simulink model "cob4_5"  (R2016a)
settings: Solver=FixedStepAuto  StartTime=0.0  StopTime=100  FixedStep=0.01  RelTol=1e-3
undefined symbols (not defined in the file): a, a2, arm_config, arm_link1, DiscIntNeverNeededParam, gripper_link, j, n, shoulder1_link, shoulder2_link, torso_link, X, Y, Z
libraries: sm_lib x81, nesl_utility x42, roblocks x3
(part 1 of 2)
settings Model: Creator=bbrito  LastModifiedBy=root

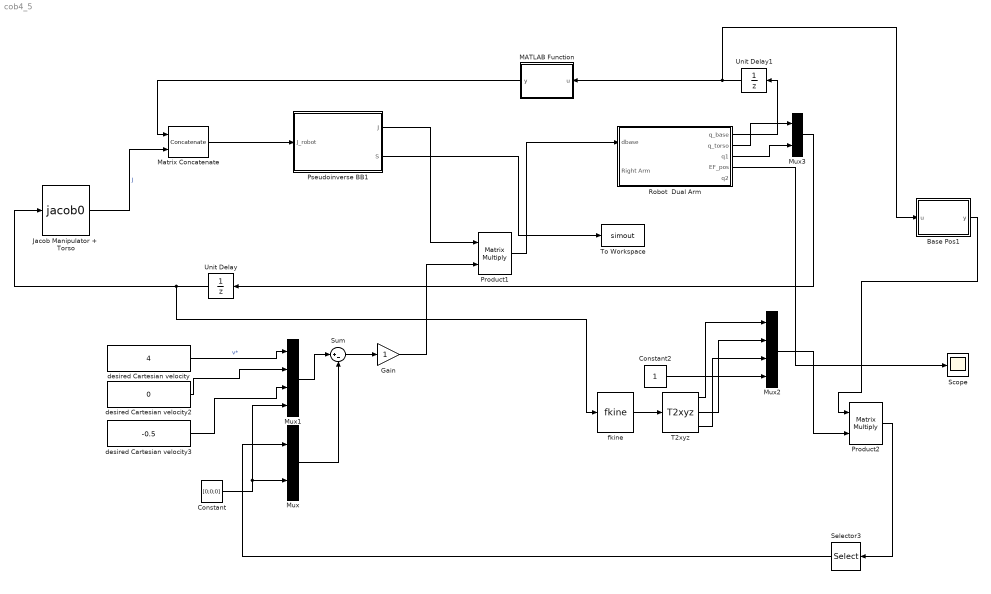
== system cob4_5 ==
  Base Pos1 : MATLAB Function  TreatAsAtomicUnit=on  mask{torso_link=torso_link}
      mask prompts: torso_link "Torso LInk"
  Constant : Constant  Value=[0;0;0]  SampleTime=-1
  Constant2 : Constant  SampleTime=-1
  Gain : Gain
  "Jacob Manipulator +  Torso " : roblocks/Kinematics/jacob0   robot=robot
  MATLAB Function : MATLAB Function  TreatAsAtomicUnit=on
  Matrix Concatenate : Concatenate  Mode=Multidimensional array  ConcatenateDimension=2
  Mux : Mux  Inputs=2
  Mux1 : Mux
  Mux2 : Mux
  Mux3 : Mux  Inputs=2
  Product1 : Product  Multiplication=Matrix(*)  SaturateOnIntegerOverflow=on  OutDataTypeStr=Inherit: Same as first input
  Product2 : Product  Multiplication=Matrix(*)  SaturateOnIntegerOverflow=on  OutDataTypeStr=Inherit: Same as first input
  Pseudoinverse BB1 : MATLAB Function  TreatAsAtomicUnit=on  mask{dim=[n(1)+4 6]}
      mask prompts: dim "Jacobian Dimensions"
  Robot  Dual Arm : Subsystem  TreatAsAtomicUnit=on
  Scope : Scope
  Selector3 : Selector  InputPortWidth=4  IndexOptions=Index vector (dialog)  Indices=[1:3]  OutputSizes=1
  Sum : Sum  Inputs=|+-
  T2xyz : roblocks/Transform Conversion/T2xyz
  To Workspace : ToWorkspace  VariableName=simout  SaveFormat=Structure  SampleTime=-1
  Unit Delay : UnitDelay  InitialCondition=zeros(n(1)+2,1)  SampleTime=-1
  Unit Delay1 : UnitDelay  InitialCondition=zeros(2,1)  SampleTime=-1
  desired Cartesian velocity : Constant  Value=4  VectorParams1D=off  SampleTime=-1
  desired Cartesian velocity2 : Constant  Value=0  VectorParams1D=off  SampleTime=-1
  desired Cartesian velocity3 : Constant  Value=-0.5  VectorParams1D=off  SampleTime=-1
  fkine : roblocks/Kinematics/fkine  robot=robot
  wires:
  fkine/1 -> T2xyz/1
  Sum/1 -> Gain/1
  Mux/1 -> Sum/2
  T2xyz/1 -> Mux2/1
  Robot  Dual Arm/3(q1) -> Mux3/2
  Constant/1 -> Mux/2, Mux1/4
  T2xyz/3 -> Mux2/3
  T2xyz/2 -> Mux2/2
  desired Cartesian velocity/1 -> Mux1/1  "v*"
  Mux1/1 -> Sum/1
  Constant2/1 -> Mux2/4
  desired Cartesian velocity2/1 -> Mux1/2
  desired Cartesian velocity3/1 -> Mux1/3
  Mux2/1 -> Product2/2
  "Jacob Manipulator +  Torso "/1 -> Matrix Concatenate/2  "J"
  Matrix Concatenate/1 -> Pseudoinverse BB1/1(J_robot)
  MATLAB Function/1(y) -> Matrix Concatenate/1
  Base Pos1/1(y) -> Product2/1
  Product2/1 -> Selector3/1
  Selector3/1 -> Mux/1
  Pseudoinverse BB1/1(J) -> Product1/1
  Gain/1 -> Product1/2
  Robot  Dual Arm/2(q_torso) -> Mux3/1
  Unit Delay/1 -> fkine/1, "Jacob Manipulator +  Torso "/1
  Mux3/1 -> Unit Delay/1
  Robot  Dual Arm/1(q_base) -> Unit Delay1/1
  Unit Delay1/1 -> Base Pos1/1(u), MATLAB Function/1(u)
  Product1/1 -> Robot  Dual Arm/1(dbase)
  Robot  Dual Arm/4(EF_pos) -> Scope/1
  Pseudoinverse BB1/2(S) -> To Workspace/1

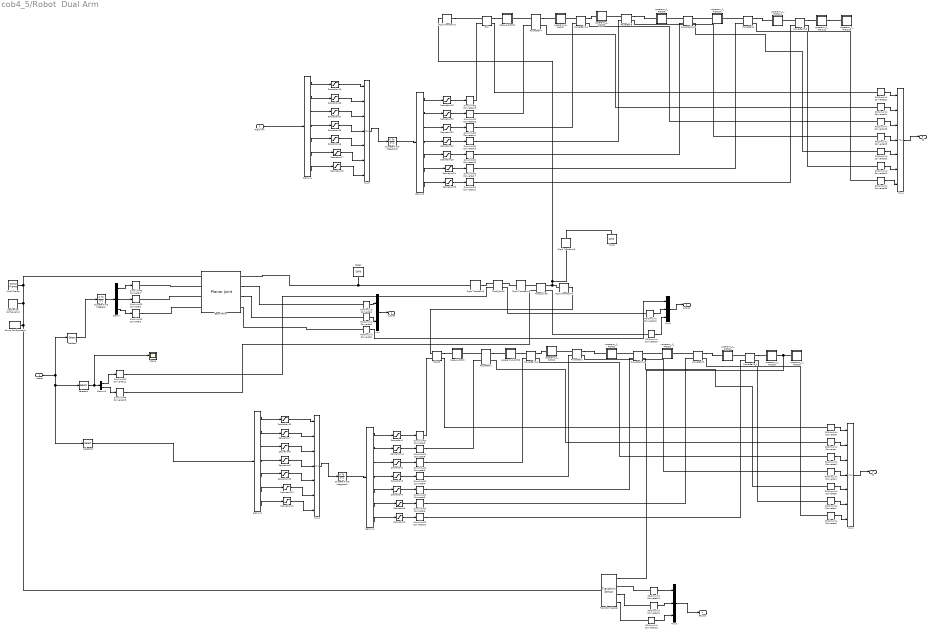
== system cob4_5/Robot  Dual Arm ==
  dbase : Inport
  Right Arm : Inport  Port=2
  Base Motion : sm_lib/Joints/Planar Joint  SenseConstraintForce=off  SenseConstraintForceX=off  SenseConstraintForceY=off  SenseConstraintForceZ=off  SenseConstraintTorque=off  SenseConstraintTorqueX=off  SenseConstraintTorqueY=off  SenseConstraintTorqueZ=off  SenseTotalForce=off  SenseTotalForceX=off  SenseTotalForceY=off  SenseTotalForceZ=off  SenseTotalTorque=off  SenseTotalTorqueX=off  SenseTotalTorqueY=off  SenseTotalTorqueZ=off  CompositeWrenchDir=FollowerOnBase  CompositeWrenchFrame=BaseFrame  PxEquilibriumPosition=0  PxEquilibriumPositionUnits=m  PxSpringStiffness=0  PxSpringStiffnessUnits=N/m  PxDampingCoefficient=0  PxDampingCoefficientUnits=N/(m/s)  PxTorqueActuationMode=ComputedTorque  PxMotionActuationMode=InputMotion  PxSensePosition=on  PxSenseVelocity=off  PxSenseAcceleration=off  PxSenseTorqueForce=off  PxPositionTargetSpecify=off  PxPositionTargetPriority=High  PxPositionTargetValue=0  PxPositionTargetValueUnits=m  PxVelocityTargetSpecify=off  PxVelocityTargetPriority=High  PxVelocityTargetValue=0  PxVelocityTargetValueUnits=m/s  PyEquilibriumPosition=0  PyEquilibriumPositionUnits=m  PySpringStiffness=0  PySpringStiffnessUnits=N/m  PyDampingCoefficient=0  PyDampingCoefficientUnits=N/(m/s)  PyTorqueActuationMode=ComputedTorque  PyMotionActuationMode=InputMotion  PySensePosition=on  PySenseVelocity=off  PySenseAcceleration=off  PySenseTorqueForce=off  PyPositionTargetSpecify=off  PyPositionTargetPriority=High  PyPositionTargetValue=0  PyPositionTargetValueUnits=m  PyVelocityTargetSpecify=off  PyVelocityTargetPriority=High  PyVelocityTargetValue=0  PyVelocityTargetValueUnits=m/s  RzEquilibriumPosition=0  RzEquilibriumPositionUnits=deg  RzSpringStiffness=0  RzSpringStiffnessUnits=N*m/deg  RzDampingCoefficient=0  RzDampingCoefficientUnits=N*m/(deg/s)  RzTorqueActuationMode=ComputedTorque  RzMotionActuationMode=InputMotion  RzSensePosition=on  RzSenseVelocity=off  RzSenseAcceleration=off  RzSenseTorqueForce=off  RzPositionTargetSpecify=off  RzPositionTargetPriority=High  RzPositionTargetValue=0  RzPositionTargetValueUnits=deg  RzVelocityTargetSpecify=off  RzVelocityTargetPriority=High  RzVelocityTargetValue=0  RzVelocityTargetValueUnits=deg/s
  Base1 : sm_lib/Body Elements/Solid  InertiaType=Custom  Mass=50  MassUnits=kg  CenterOfMass=[0 0 0]  CenterOfMassUnits=m  MomentsOfInertia=[5.652232699207 5.669473158652 3.683196351726]  MomentsOfInertiaUnits=kg*m^2  ProductsOfInertia=[-0.009719934438 1.293988226423 -0.007379583694]  ProductsOfInertiaUnits=kg*m^2  DensityBased=on  Density=1000  DensityUnits=kg/(m^3)  DoExposeReferenceFrame=on  SerializedFrames=<Frames/>  GraphicType=FromGeometry  MarkerShape=Sphere  MarkerSize=10  GraphicVisPropType=SimpleVisualProperties  GraphicDiffuseColor=[0.5 0.5 0.5]  GraphicSpecularColor=[0.5 0.5 0.5 1.0]  GraphicAmbientColor=[0.15 0.15 0.15 1.0]  GraphicEmissiveColor=[0.0 0.0 0.0 1.0]  GraphicShininess=75  GraphicOpacity=1.0  GeometryShape=FromFile  RectangleSize=[1 1]  RectangleSizeUnits=m  BrickDimensions=[1 1 1]  BrickDimensionUnits=m  CylinderRadius=1  CylinderRadiusUnits=m  CylinderLength=1  CylinderLengthUnits=m  SphereRadius=1  SphereRadiusUnits=m  EllipsoidRadii=[1 1 1]  EllipsoidRadiiUnits=m  ExtrusionCrossSection=[1 1; -1 1; -1 -1; 1 -1]  ExtrusionCrossSectionUnits=m  ExtrusionLength=1  ExtrusionLengthUnits=m  PolygonNumSides=3  PolygonOuterRadius=1  PolygonOuterRadiusUnits=m  ExtGeomFileType=STL  ExtGeomFileName=/home/bbrito/schunk_sim/base.stl  ExtGeomFileUnits=m  RevolutionCrossSection=[1 1; 1 -1; 2 -1; 2 1]  RevolutionCrossSectionUnits=m  RevolutionExtent=Full  RevolutionAngle=180  RevolutionAngleUnits=deg
  DL1 : sm_lib/Joints/Revolute Joint  SenseConstraintForce=off  SenseConstraintForceX=off  SenseConstraintForceY=off  SenseConstraintForceZ=off  SenseConstraintTorque=off  SenseConstraintTorqueX=off  SenseConstraintTorqueY=off  SenseConstraintTorqueZ=off  SenseTotalForce=off  SenseTotalForceX=off  SenseTotalForceY=off  SenseTotalForceZ=off  SenseTotalTorque=off  SenseTotalTorqueX=off  SenseTotalTorqueY=off  SenseTotalTorqueZ=off  CompositeWrenchDir=FollowerOnBase  CompositeWrenchFrame=BaseFrame  EquilibriumPosition=0  EquilibriumPositionUnits=deg  SpringStiffness=0  SpringStiffnessUnits=N*m/deg  DampingCoefficient=0  DampingCoefficientUnits=N*m/(deg/s)  TorqueActuationMode=ComputedTorque  MotionActuationMode=InputMotion  SensePosition=on  SenseVelocity=off  SenseAcceleration=off  SenseTorqueForce=off  PositionTargetSpecify=on  PositionTargetPriority=High  PositionTargetValue=0  PositionTargetValueUnits=deg  VelocityTargetSpecify=on  VelocityTargetPriority=High  VelocityTargetValue=0  VelocityTargetValueUnits=deg/s
  DL100 : sm_lib/Joints/Revolute Joint  SenseConstraintForce=off  SenseConstraintForceX=off  SenseConstraintForceY=off  SenseConstraintForceZ=off  SenseConstraintTorque=off  SenseConstraintTorqueX=off  SenseConstraintTorqueY=off  SenseConstraintTorqueZ=off  SenseTotalForce=off  SenseTotalForceX=off  SenseTotalForceY=off  SenseTotalForceZ=off  SenseTotalTorque=off  SenseTotalTorqueX=off  SenseTotalTorqueY=off  SenseTotalTorqueZ=off  CompositeWrenchDir=FollowerOnBase  CompositeWrenchFrame=BaseFrame  EquilibriumPosition=0  EquilibriumPositionUnits=deg  SpringStiffness=0  SpringStiffnessUnits=N*m/deg  DampingCoefficient=0  DampingCoefficientUnits=N*m/(deg/s)  TorqueActuationMode=ComputedTorque  MotionActuationMode=InputMotion  SensePosition=on  SenseVelocity=off  SenseAcceleration=off  SenseTorqueForce=off  PositionTargetSpecify=on  PositionTargetPriority=High  PositionTargetValue=0  PositionTargetValueUnits=deg  VelocityTargetSpecify=on  VelocityTargetPriority=High  VelocityTargetValue=0  VelocityTargetValueUnits=deg/s
  Demux : Demux  Outputs=3
  Demux{1..4} (4 alike) : Demux  Outputs=n(1)-1
  Demux5 : Demux  Outputs=2
  Discrete-Time Integrator : DiscreteIntegrator  InitialCondition=[0;0;0]  InitialConditionSetting=State (most efficient)  SampleTime=-1  ICPrevOutput=DiscIntNeverNeededParam  ICPrevScaledInput=DiscIntNeverNeededParam
  Discrete-Time Integrator1 : DiscreteIntegrator  InitialCondition=zeros(n(1)-1,1)  InitialConditionSetting=State (most efficient)  SampleTime=-1  ICPrevOutput=DiscIntNeverNeededParam  ICPrevScaledInput=DiscIntNeverNeededParam
  Discrete-Time Integrator3 : DiscreteIntegrator  InitialCondition=zeros(n(1)-1,1)  InitialConditionSetting=State (most efficient)  SampleTime=-1  ICPrevOutput=DiscIntNeverNeededParam  ICPrevScaledInput=DiscIntNeverNeededParam
  Mechanism Configuration : sm_lib/Utilities/Mechanism Configuration  UniformGravity=Constant  GravityVector=[0 0 -9.81]  GravityUnits=m/s^2  LinearizationDelta=0.01
  Mux : Mux  Inputs=2
  Mux{1..2,4..5} (4 alike) : Mux  Inputs=n(1)-1
  Mux3 : Mux  Inputs=3
  Mux6 : Mux  Inputs=3
  PS-Simulink Converter{,1..15,18..23} (22 alike) : nesl_utility/PS-Simulink Converter  PhysicalDomain=network_engine_domain  SubClassName=ps_output  LeftPortType=input  RightPortType=output  PseudoPeriodic=off  Frequencies=[]  Unit=1  AffineConversion=off
  PowerBall{1..6} (6 alike) : sm_lib/Joints/Revolute Joint  SenseConstraintForce=off  SenseConstraintForceX=off  SenseConstraintForceY=off  SenseConstraintForceZ=off  SenseConstraintTorque=off  SenseConstraintTorqueX=off  SenseConstraintTorqueY=off  SenseConstraintTorqueZ=off  SenseTotalForce=off  SenseTotalForceX=off  SenseTotalForceY=off  SenseTotalForceZ=off  SenseTotalTorque=off  SenseTotalTorqueX=off  SenseTotalTorqueY=off  SenseTotalTorqueZ=off  CompositeWrenchDir=FollowerOnBase  CompositeWrenchFrame=BaseFrame  EquilibriumPosition=0  EquilibriumPositionUnits=deg  SpringStiffness=0  SpringStiffnessUnits=N*m/deg  DampingCoefficient=0  DampingCoefficientUnits=N*m/(deg/s)  TorqueActuationMode=ComputedTorque  MotionActuationMode=InputMotion  SensePosition=on  SenseVelocity=off  SenseAcceleration=off  SenseTorqueForce=off  PositionTargetSpecify=on  PositionTargetPriority=High  PositionTargetValue=0  PositionTargetValueUnits=deg  VelocityTargetSpecify=on  VelocityTargetPriority=High  VelocityTargetValue=0  VelocityTargetValueUnits=deg/s
  PowerBall1_1 : sm_lib/Joints/Revolute Joint  SenseConstraintForce=off  SenseConstraintForceX=off  SenseConstraintForceY=off  SenseConstraintForceZ=off  SenseConstraintTorque=off  SenseConstraintTorqueX=off  SenseConstraintTorqueY=off  SenseConstraintTorqueZ=off  SenseTotalForce=off  SenseTotalForceX=off  SenseTotalForceY=off  SenseTotalForceZ=off  SenseTotalTorque=off  SenseTotalTorqueX=off  SenseTotalTorqueY=off  SenseTotalTorqueZ=off  CompositeWrenchDir=FollowerOnBase  CompositeWrenchFrame=BaseFrame  EquilibriumPosition=0  EquilibriumPositionUnits=deg  SpringStiffness=0  SpringStiffnessUnits=N*m/deg  DampingCoefficient=0  DampingCoefficientUnits=N*m/(deg/s)  TorqueActuationMode=ComputedTorque  MotionActuationMode=InputMotion  SensePosition=on  SenseVelocity=off  SenseAcceleration=off  SenseTorqueForce=off  PositionTargetSpecify=on  PositionTargetPriority=High  PositionTargetValue=0  PositionTargetValueUnits=deg  VelocityTargetSpecify=on  VelocityTargetPriority=High  VelocityTargetValue=0  VelocityTargetValueUnits=deg/s
  PowerBall1_2 : sm_lib/Joints/Revolute Joint  SenseConstraintForce=off  SenseConstraintForceX=off  SenseConstraintForceY=off  SenseConstraintForceZ=off  SenseConstraintTorque=off  SenseConstraintTorqueX=off  SenseConstraintTorqueY=off  SenseConstraintTorqueZ=off  SenseTotalForce=off  SenseTotalForceX=off  SenseTotalForceY=off  SenseTotalForceZ=off  SenseTotalTorque=off  SenseTotalTorqueX=off  SenseTotalTorqueY=off  SenseTotalTorqueZ=off  CompositeWrenchDir=FollowerOnBase  CompositeWrenchFrame=BaseFrame  EquilibriumPosition=0  EquilibriumPositionUnits=deg  SpringStiffness=0  SpringStiffnessUnits=N*m/deg  DampingCoefficient=0  DampingCoefficientUnits=N*m/(deg/s)  TorqueActuationMode=ComputedTorque  MotionActuationMode=InputMotion  SensePosition=on  SenseVelocity=off  SenseAcceleration=off  SenseTorqueForce=off  PositionTargetSpecify=on  PositionTargetPriority=High  PositionTargetValue=0  PositionTargetValueUnits=deg  VelocityTargetSpecify=on  VelocityTargetPriority=High  VelocityTargetValue=0  VelocityTargetValueUnits=deg/s
  PowerBall2_1 : sm_lib/Joints/Revolute Joint  SenseConstraintForce=off  SenseConstraintForceX=off  SenseConstraintForceY=off  SenseConstraintForceZ=off  SenseConstraintTorque=off  SenseConstraintTorqueX=off  SenseConstraintTorqueY=off  SenseConstraintTorqueZ=off  SenseTotalForce=off  SenseTotalForceX=off  SenseTotalForceY=off  SenseTotalForceZ=off  SenseTotalTorque=off  SenseTotalTorqueX=off  SenseTotalTorqueY=off  SenseTotalTorqueZ=off  CompositeWrenchDir=FollowerOnBase  CompositeWrenchFrame=BaseFrame  EquilibriumPosition=0  EquilibriumPositionUnits=deg  SpringStiffness=0  SpringStiffnessUnits=N*m/deg  DampingCoefficient=0  DampingCoefficientUnits=N*m/(deg/s)  TorqueActuationMode=ComputedTorque  MotionActuationMode=InputMotion  SensePosition=on  SenseVelocity=off  SenseAcceleration=off  SenseTorqueForce=off  PositionTargetSpecify=on  PositionTargetPriority=High  PositionTargetValue=0  PositionTargetValueUnits=deg  VelocityTargetSpecify=on  VelocityTargetPriority=High  VelocityTargetValue=0  VelocityTargetValueUnits=deg/s
  PowerBall2_2 : sm_lib/Joints/Revolute Joint  SenseConstraintForce=off  SenseConstraintForceX=off  SenseConstraintForceY=off  SenseConstraintForceZ=off  SenseConstraintTorque=off  SenseConstraintTorqueX=off  SenseConstraintTorqueY=off  SenseConstraintTorqueZ=off  SenseTotalForce=off  SenseTotalForceX=off  SenseTotalForceY=off  SenseTotalForceZ=off  SenseTotalTorque=off  SenseTotalTorqueX=off  SenseTotalTorqueY=off  SenseTotalTorqueZ=off  CompositeWrenchDir=FollowerOnBase  CompositeWrenchFrame=BaseFrame  EquilibriumPosition=0  EquilibriumPositionUnits=deg  SpringStiffness=0  SpringStiffnessUnits=N*m/deg  DampingCoefficient=0  DampingCoefficientUnits=N*m/(deg/s)  TorqueActuationMode=ComputedTorque  MotionActuationMode=InputMotion  SensePosition=on  SenseVelocity=off  SenseAcceleration=off  SenseTorqueForce=off  PositionTargetSpecify=on  PositionTargetPriority=High  PositionTargetValue=0  PositionTargetValueUnits=deg  VelocityTargetSpecify=on  VelocityTargetPriority=High  VelocityTargetValue=0  VelocityTargetValueUnits=deg/s
  PowerBall3_1 : sm_lib/Joints/Revolute Joint  SenseConstraintForce=off  SenseConstraintForceX=off  SenseConstraintForceY=off  SenseConstraintForceZ=off  SenseConstraintTorque=off  SenseConstraintTorqueX=off  SenseConstraintTorqueY=off  SenseConstraintTorqueZ=off  SenseTotalForce=off  SenseTotalForceX=off  SenseTotalForceY=off  SenseTotalForceZ=off  SenseTotalTorque=off  SenseTotalTorqueX=off  SenseTotalTorqueY=off  SenseTotalTorqueZ=off  CompositeWrenchDir=FollowerOnBase  CompositeWrenchFrame=BaseFrame  EquilibriumPosition=0  EquilibriumPositionUnits=deg  SpringStiffness=0  SpringStiffnessUnits=N*m/deg  DampingCoefficient=0  DampingCoefficientUnits=N*m/(deg/s)  TorqueActuationMode=ComputedTorque  MotionActuationMode=InputMotion  SensePosition=on  SenseVelocity=off  SenseAcceleration=off  SenseTorqueForce=off  PositionTargetSpecify=on  PositionTargetPriority=High  PositionTargetValue=0  PositionTargetValueUnits=deg  VelocityTargetSpecify=on  VelocityTargetPriority=High  VelocityTargetValue=0  VelocityTargetValueUnits=deg/s
  PowerBall3_2 : sm_lib/Joints/Revolute Joint  SenseConstraintForce=off  SenseConstraintForceX=off  SenseConstraintForceY=off  SenseConstraintForceZ=off  SenseConstraintTorque=off  SenseConstraintTorqueX=off  SenseConstraintTorqueY=off  SenseConstraintTorqueZ=off  SenseTotalForce=off  SenseTotalForceX=off  SenseTotalForceY=off  SenseTotalForceZ=off  SenseTotalTorque=off  SenseTotalTorqueX=off  SenseTotalTorqueY=off  SenseTotalTorqueZ=off  CompositeWrenchDir=FollowerOnBase  CompositeWrenchFrame=BaseFrame  EquilibriumPosition=0  EquilibriumPositionUnits=deg  SpringStiffness=0  SpringStiffnessUnits=N*m/deg  DampingCoefficient=0  DampingCoefficientUnits=N*m/(deg/s)  TorqueActuationMode=ComputedTorque  MotionActuationMode=InputMotion  SensePosition=on  SenseVelocity=off  SenseAcceleration=off  SenseTorqueForce=off  PositionTargetSpecify=on  PositionTargetPriority=High  PositionTargetValue=0  PositionTargetValueUnits=deg  VelocityTargetSpecify=on  VelocityTargetPriority=High  VelocityTargetValue=0  VelocityTargetValueUnits=deg/s
  Rigid Transform1 : sm_lib/Frames and Transforms/Rigid Transform  TranslationMethod=Cartesian  TranslationLengthUnit=m  TranslationStandardAxis=+Z  TranslationStandardOffset=0  TranslationCartesianOffset=a2(1:3,4,1)  TranslationROffset=0  TranslationROffsetUnits=m  TranslationZOffset=0  TranslationZOffsetUnits=m  TranslationThetaOffset=0  TranslationThetaOffsetUnits=deg  RotationMethod=RotationMatrix  RotationAngleUnits=deg  RotationStandardAxis=+Z  RotationAngle=0.0  RotationArbitraryAxis=[0 0 1]  FollAlignAxisA=+X  BaseAlignAxisA=+Y  FollAlignAxisB=+Y  BaseAlignAxisB=+Z  RotationSequenceAxes=FollowerAxes  RotationSequence=XYX  RotationSequenceAngles=[0 0 0]  RotationSequenceAnglesUnits=deg  RotationMatrix=a2(1:3,1:3,1)
  Rigid Transform2 : sm_lib/Frames and Transforms/Rigid Transform  TranslationMethod=Cartesian  TranslationLengthUnit=m  TranslationStandardAxis=+Z  TranslationStandardOffset=0  TranslationCartesianOffset=a(1:3,4,2+j)  TranslationROffset=0  TranslationROffsetUnits=m  TranslationZOffset=0  TranslationZOffsetUnits=m  TranslationThetaOffset=0  TranslationThetaOffsetUnits=deg  RotationMethod=RotationMatrix  RotationAngleUnits=deg  RotationStandardAxis=+Z  RotationAngle=0.0  RotationArbitraryAxis=[0 0 1]  FollAlignAxisA=+X  BaseAlignAxisA=+Y  FollAlignAxisB=+Y  BaseAlignAxisB=+Z  RotationSequenceAxes=FollowerAxes  RotationSequence=XYX  RotationSequenceAngles=[0 0 0]  RotationSequenceAnglesUnits=deg  RotationMatrix=a(1:3,1:3,2+j)
  Rigid Transform3 : sm_lib/Frames and Transforms/Rigid Transform  TranslationMethod=Cartesian  TranslationLengthUnit=m  TranslationStandardAxis=+Z  TranslationStandardOffset=0  TranslationCartesianOffset=a(1:3,4,3+j)  TranslationROffset=0  TranslationROffsetUnits=m  TranslationZOffset=0  TranslationZOffsetUnits=m  TranslationThetaOffset=0  TranslationThetaOffsetUnits=deg  RotationMethod=RotationMatrix  RotationAngleUnits=deg  RotationStandardAxis=+Z  RotationAngle=0.0  RotationArbitraryAxis=[0 0 1]  FollAlignAxisA=+X  BaseAlignAxisA=+Y  FollAlignAxisB=+Y  BaseAlignAxisB=+Z  RotationSequenceAxes=FollowerAxes  RotationSequence=XYX  RotationSequenceAngles=[0 0 0]  RotationSequenceAnglesUnits=deg  RotationMatrix=a(1:3,1:3,3+j)
  Rigid Transform4 : sm_lib/Frames and Transforms/Rigid Transform  TranslationMethod=Cartesian  TranslationLengthUnit=m  TranslationStandardAxis=+Z  TranslationStandardOffset=0  TranslationCartesianOffset=a(1:3,4,4+j)  TranslationROffset=0  TranslationROffsetUnits=m  TranslationZOffset=0  TranslationZOffsetUnits=m  TranslationThetaOffset=0  TranslationThetaOffsetUnits=deg  RotationMethod=RotationMatrix  RotationAngleUnits=deg  RotationStandardAxis=+Z  RotationAngle=0.0  RotationArbitraryAxis=[0 0 1]  FollAlignAxisA=+X  BaseAlignAxisA=+Y  FollAlignAxisB=+Y  BaseAlignAxisB=+Z  RotationSequenceAxes=FollowerAxes  RotationSequence=XYX  RotationSequenceAngles=[0 0 0]  RotationSequenceAnglesUnits=deg  RotationMatrix=a(1:3,1:3,4+j)
  Rigid Transform5 : sm_lib/Frames and Transforms/Rigid Transform  TranslationMethod=Cartesian  TranslationLengthUnit=m  TranslationStandardAxis=+Z  TranslationStandardOffset=0  TranslationCartesianOffset=torso_link(1:3,4,1)  TranslationROffset=0  TranslationROffsetUnits=m  TranslationZOffset=0  TranslationZOffsetUnits=m  TranslationThetaOffset=0  TranslationThetaOffsetUnits=deg  RotationMethod=RotationMatrix  RotationAngleUnits=deg  RotationStandardAxis=+Z  RotationAngle=0.0  RotationArbitraryAxis=[0 0 1]  FollAlignAxisA=+X  BaseAlignAxisA=+Y  FollAlignAxisB=+Y  BaseAlignAxisB=+Z  RotationSequenceAxes=FollowerAxes  RotationSequence=XYX  RotationSequenceAngles=[0 0 0]  RotationSequenceAnglesUnits=deg  RotationMatrix=torso_link(1:3,1:3,1)
  Saturation1 : Saturate  UpperLimit=arm_config.joint.limits(1)  LowerLimit=arm_config.joint.limits(2)
  Saturation10 : Saturate  UpperLimit=arm_config.joint.speed_limits(5)  LowerLimit=-arm_config.joint.speed_limits(5)
  Saturation11 : Saturate  UpperLimit=arm_config.joint.speed_limits(6)  LowerLimit=-arm_config.joint.speed_limits(6)
  Saturation12 : Saturate  UpperLimit=arm_config.joint.speed_limits(7)  LowerLimit=-arm_config.joint.speed_limits(7)
  Saturation13 : Saturate  UpperLimit=arm_config.joint.speed_limits(1)  LowerLimit=-arm_config.joint.speed_limits(1)
  Saturation14 : Saturate  UpperLimit=arm_config.joint.limits(3)  LowerLimit=arm_config.joint.limits(4)
  Saturation15 : Saturate  UpperLimit=arm_config.joint.limits(1)  LowerLimit=arm_config.joint.limits(2)
  Saturation16 : Saturate  UpperLimit=arm_config.joint.speed_limits(5)  LowerLimit=-arm_config.joint.speed_limits(5)
  Saturation17 : Saturate  UpperLimit=arm_config.joint.speed_limits(6)  LowerLimit=-arm_config.joint.speed_limits(6)
  Saturation18 : Saturate  UpperLimit=arm_config.joint.speed_limits(7)  LowerLimit=-arm_config.joint.speed_limits(7)
  Saturation19 : Saturate  UpperLimit=arm_config.joint.speed_limits(1)  LowerLimit=-arm_config.joint.speed_limits(1)
  Saturation2 : Saturate  UpperLimit=arm_config.joint.limits(5)  LowerLimit=arm_config.joint.limits(6)
  Saturation20 : Saturate  UpperLimit=arm_config.joint.limits(3)  LowerLimit=arm_config.joint.limits(4)
  Saturation21 : Saturate  UpperLimit=arm_config.joint.limits(5)  LowerLimit=arm_config.joint.limits(6)
  Saturation22 : Saturate  UpperLimit=arm_config.joint.limits(7)  LowerLimit=arm_config.joint.limits(8)
  Saturation23 : Saturate  UpperLimit=arm_config.joint.limits(9)  LowerLimit=arm_config.joint.limits(10)
  Saturation24 : Saturate  UpperLimit=arm_config.joint.limits(11)  LowerLimit=arm_config.joint.limits(12)
  Saturation25 : Saturate  UpperLimit=arm_config.joint.limits(13)  LowerLimit=arm_config.joint.limits(14)
  Saturation26 : Saturate  UpperLimit=arm_config.joint.speed_limits(2)  LowerLimit=-arm_config.joint.speed_limits(2)
  Saturation27 : Saturate  UpperLimit=arm_config.joint.speed_limits(3)  LowerLimit=-arm_config.joint.speed_limits(3)
  Saturation28 : Saturate  UpperLimit=arm_config.joint.speed_limits(4)  LowerLimit=-arm_config.joint.speed_limits(4)
  Saturation3 : Saturate  UpperLimit=arm_config.joint.limits(7)  LowerLimit=arm_config.joint.limits(8)
  Saturation4 : Saturate  UpperLimit=arm_config.joint.limits(9)  LowerLimit=arm_config.joint.limits(10)
  Saturation5 : Saturate  UpperLimit=arm_config.joint.limits(11)  LowerLimit=arm_config.joint.limits(12)
  Saturation6 : Saturate  UpperLimit=arm_config.joint.limits(13)  LowerLimit=arm_config.joint.limits(14)
  Saturation7 : Saturate  UpperLimit=arm_config.joint.speed_limits(2)  LowerLimit=-arm_config.joint.speed_limits(2)
  Saturation8 : Saturate  UpperLimit=arm_config.joint.speed_limits(3)  LowerLimit=-arm_config.joint.speed_limits(3)
  Saturation9 : Saturate  UpperLimit=arm_config.joint.speed_limits(4)  LowerLimit=-arm_config.joint.speed_limits(4)
  Scope : Scope
  Selector : Selector  InputPortWidth=n(1)+4  IndexOptions=Index vector (dialog)  Indices=[1:3]  OutputSizes=1
  Selector1 : Selector  InputPortWidth=n(1)+4  IndexOptions=Index vector (dialog)  Indices=[4:5]  OutputSizes=1
  Selector2 : Selector  InputPortWidth=n(1)+4  IndexOptions=Index vector (dialog)  Indices=[6:12]  OutputSizes=1
  Simulink-PS Converter{1..19} (19 alike) : nesl_utility/Simulink-PS Converter  PhysicalDomain=network_engine_domain  SubClassName=ps_input  LeftPortType=input  RightPortType=output  PseudoPeriodic=off  Frequencies=[]  NoiseDistribution=none  NoiseParameters=[]  Unit=1  AffineConversion=off  InputFiltering=off  SimscapeFilterOrder=1  InputFilterTimeConstant=0.001  UdotUserProvided=1
  Solver Configuration : nesl_utility/Solver Configuration  PhysicalDomain=network_engine_domain  SubClassName=solver  LeftPortType=input  RightPortType=generic  Accelerate=off  Tones=[]  Harmonics=[]  SimulateNoise=off  Profile=off  UseLocalSampling=off  EnableSwitchedLinearOptims=on  FrequencyDomain=off  UseCCode=off  RelTol=0.001  AbsTol=1e-06  MinStep=1e-09  ToWorkspace=off  RevertToSquareIcSolve=off  NumHomotopyIterations=100  PhasorMode=off  PhasorModeNumHarmonics=1  OverrideAbsTol=off  DoDC=off  ResidualTolerance=1e-06  UseLocalSolver=on  LocalSolverChoice=NE_BACKWARD_EULER_ADVANCER  LocalSolverSampleTime=0.01  DoFixedCost=on  MaxNonlinIter=3  MaxModeIter=2  LinearAlgebra=Full  DelaysMemoryBudget=1024  AutomaticFiltering=off  FilteringTimeConstant=0.001
  Torso : sm_lib/Body Elements/Solid  InertiaType=Custom  Mass=5  MassUnits=kg  CenterOfMass=[0 0 0]  CenterOfMassUnits=m  MomentsOfInertia=[1 1 1]  MomentsOfInertiaUnits=kg*m^2  ProductsOfInertia=[0 0 0]  ProductsOfInertiaUnits=kg*m^2  DensityBased=on  Density=1000  DensityUnits=kg/(m^3)  DoExposeReferenceFrame=on  SerializedFrames=<Frames/>  GraphicType=FromGeometry  MarkerShape=Sphere  MarkerSize=10  GraphicVisPropType=SimpleVisualProperties  GraphicDiffuseColor=[0.5 0.5 0.5]  GraphicSpecularColor=[0.5 0.5 0.5 1.0]  GraphicAmbientColor=[0.15 0.15 0.15 1.0]  GraphicEmissiveColor=[0.0 0.0 0.0 1.0]  GraphicShininess=75  GraphicOpacity=1.0  GeometryShape=FromFile  RectangleSize=[1 1]  RectangleSizeUnits=m  BrickDimensions=[1 1 1]  BrickDimensionUnits=m  CylinderRadius=1  CylinderRadiusUnits=m  CylinderLength=1  CylinderLengthUnits=m  SphereRadius=1  SphereRadiusUnits=m  EllipsoidRadii=[1 1 1]  EllipsoidRadiiUnits=m  ExtrusionCrossSection=[1 1; -1 1; -1 -1; 1 -1]  ExtrusionCrossSectionUnits=m  ExtrusionLength=1  ExtrusionLengthUnits=m  PolygonNumSides=3  PolygonOuterRadius=1  PolygonOuterRadiusUnits=m  ExtGeomFileType=STL  ExtGeomFileName=/home/bbrito/schunk_sim/torso.stl  ExtGeomFileUnits=m  RevolutionCrossSection=[1 1; 1 -1; 2 -1; 2 1]  RevolutionCrossSectionUnits=m  RevolutionExtent=Full  RevolutionAngle=180  RevolutionAngleUnits=deg
  Torso_Joint2 : sm_lib/Joints/Revolute Joint  SenseConstraintForce=off  SenseConstraintForceX=off  SenseConstraintForceY=off  SenseConstraintForceZ=off  SenseConstraintTorque=off  SenseConstraintTorqueX=off  SenseConstraintTorqueY=off  SenseConstraintTorqueZ=off  SenseTotalForce=off  SenseTotalForceX=off  SenseTotalForceY=off  SenseTotalForceZ=off  SenseTotalTorque=off  SenseTotalTorqueX=off  SenseTotalTorqueY=off  SenseTotalTorqueZ=off  CompositeWrenchDir=FollowerOnBase  CompositeWrenchFrame=BaseFrame  EquilibriumPosition=0  EquilibriumPositionUnits=deg  SpringStiffness=0  SpringStiffnessUnits=N*m/deg  DampingCoefficient=0  DampingCoefficientUnits=N*m/(deg/s)  TorqueActuationMode=ComputedTorque  MotionActuationMode=InputMotion  SensePosition=on  SenseVelocity=off  SenseAcceleration=off  SenseTorqueForce=off  PositionTargetSpecify=on  PositionTargetPriority=High  PositionTargetValue=0  PositionTargetValueUnits=deg  VelocityTargetSpecify=on  VelocityTargetPriority=High  VelocityTargetValue=0  VelocityTargetValueUnits=deg/s
  Torso_Joint3 : sm_lib/Joints/Revolute Joint  SenseConstraintForce=off  SenseConstraintForceX=off  SenseConstraintForceY=off  SenseConstraintForceZ=off  SenseConstraintTorque=off  SenseConstraintTorqueX=off  SenseConstraintTorqueY=off  SenseConstraintTorqueZ=off  SenseTotalForce=off  SenseTotalForceX=off  SenseTotalForceY=off  SenseTotalForceZ=off  SenseTotalTorque=off  SenseTotalTorqueX=off  SenseTotalTorqueY=off  SenseTotalTorqueZ=off  CompositeWrenchDir=FollowerOnBase  CompositeWrenchFrame=BaseFrame  EquilibriumPosition=0  EquilibriumPositionUnits=deg  SpringStiffness=0  SpringStiffnessUnits=N*m/deg  DampingCoefficient=0  DampingCoefficientUnits=N*m/(deg/s)  TorqueActuationMode=ComputedTorque  MotionActuationMode=InputMotion  SensePosition=on  SenseVelocity=off  SenseAcceleration=off  SenseTorqueForce=off  PositionTargetSpecify=on  PositionTargetPriority=High  PositionTargetValue=0  PositionTargetValueUnits=deg  VelocityTargetSpecify=on  VelocityTargetPriority=High  VelocityTargetValue=0  VelocityTargetValueUnits=deg/s
  Transform Sensor : sm_lib/Frames and Transforms/Transform Sensor  MeasurementFrame=World  SenseAngle=off  SenseAxis=off  SenseAngle1=off  SenseAngle2=off  SenseAngle3=off  SenseQ=off  SenseR=off  SenseOmegaX=off  SenseOmegaY=off  SenseOmegaZ=off  SenseOmega1=off  SenseOmega2=off  SenseOmega3=off  SenseQDot=off  SenseRDot=off  SenseAlphaX=off  SenseAlphaY=off  SenseAlphaZ=off  SenseAlpha1=off  SenseAlpha2=off  SenseAlpha3=off  SenseQDDot=off  SenseRDDot=off  SenseX=on  SenseY=on  SenseZ=on  SenseRad=off  SenseAzim=off  SenseDist=off  SenseInc=off  SenseXDot=off  SenseYDot=off  SenseZDot=off  SenseRadDot=off  SenseAzimDot=off  SenseDistDot=off  SenseIncDot=off  SenseXDDot=off  SenseYDDot=off  SenseZDDot=off  SenseRadDDot=off  SenseAzimDDot=off  SenseDistDDot=off  SenseIncDDot=off
  World Frame : sm_lib/Frames and Transforms/World Frame
  base_1_RIGID : Subsystem
  base_1_RIGID1 : Subsystem
  upperarm_1_RIGID : Subsystem
  upperarm_1_RIGID1 : Subsystem
  upperarm_1_RIGID10 : Subsystem
  upperarm_1_RIGID11 : Subsystem
  upperarm_1_RIGID12 : Subsystem
  upperarm_1_RIGID13 : Subsystem
  upperarm_1_RIGID2 : Subsystem
  upperarm_1_RIGID3 : Subsystem
  upperarm_1_RIGID4 : Subsystem
  upperarm_1_RIGID5 : Subsystem
  upperarm_1_RIGID6 : Subsystem
  upperarm_1_RIGID7 : Subsystem
  upperarm_1_RIGID8 : Subsystem
  upperarm_1_RIGID9 : Subsystem
  q_base : Outport  PortDimensions=[2 1]
  q_torso : Outport  Port=2
  q1 : Outport  Port=3
  EF_pos : Outport  Port=4
  q2 : Outport  Port=5
  wires:
  Demux/2 -> Simulink-PS Converter1/1
  Demux/1 -> Simulink-PS Converter7/1
  Mux/1 -> q_base/1
  PS-Simulink Converter6/1 -> Mux/1
  PS-Simulink Converter1/1 -> Mux/2
  PS-Simulink Converter2/1 -> Mux6/1
  Discrete-Time Integrator/1 -> Demux/1
  Mux1/1 -> q1/1
  Discrete-Time Integrator1/1 -> Demux1/1
  PS-Simulink Converter8/1 -> Mux1/1
  PS-Simulink Converter/1 -> Mux1/2
  PS-Simulink Converter3/1 -> Mux1/3
  PS-Simulink Converter4/1 -> Mux1/4
  PS-Simulink Converter5/1 -> Mux1/5
  PS-Simulink Converter7/1 -> Mux1/6
  Saturation14/1 -> Simulink-PS Converter8/1
  Demux1/2 -> Saturation14/1
  Saturation2/1 -> Simulink-PS Converter3/1
  Demux1/3 -> Saturation2/1
  Saturation3/1 -> Simulink-PS Converter4/1
  Demux1/4 -> Saturation3/1
  Demux1/5 -> Saturation4/1
  Saturation4/1 -> Simulink-PS Converter5/1
  Saturation6/1 -> Simulink-PS Converter10/1
  Demux1/7 -> Saturation6/1
  Demux1/6 -> Saturation5/1
  Saturation5/1 -> Simulink-PS Converter6/1
  Demux2/2 -> Saturation7/1
  Demux2/3 -> Saturation8/1
  Demux2/4 -> Saturation9/1
  Demux2/5 -> Saturation10/1
  Demux2/7 -> Saturation12/1
  Demux2/6 -> Saturation11/1
  Saturation13/1 -> Mux2/1
  Demux2/1 -> Saturation13/1
  Demux1/1 -> Saturation1/1
  Saturation1/1 -> Simulink-PS Converter9/1
  Saturation7/1 -> Mux2/2
  Saturation8/1 -> Mux2/3
  Saturation9/1 -> Mux2/4
  Saturation10/1 -> Mux2/5
  Saturation11/1 -> Mux2/6
  Saturation12/1 -> Mux2/7
  Mux2/1 -> Discrete-Time Integrator1/1
  PS-Simulink Converter12/1 -> Mux3/2
  PS-Simulink Converter11/1 -> Mux3/1
  PS-Simulink Converter13/1 -> Mux3/3
  Mux3/1 -> EF_pos/1
  PS-Simulink Converter9/1 -> Mux1/7
  Mux4/1 -> q2/1
  Discrete-Time Integrator3/1 -> Demux3/1
  PS-Simulink Converter22/1 -> Mux4/1
  PS-Simulink Converter14/1 -> Mux4/2
  PS-Simulink Converter18/1 -> Mux4/3
  PS-Simulink Converter19/1 -> Mux4/4
  PS-Simulink Converter20/1 -> Mux4/5
  PS-Simulink Converter21/1 -> Mux4/6
  Saturation20/1 -> Simulink-PS Converter18/1
  Demux3/2 -> Saturation20/1
  Saturation21/1 -> Simulink-PS Converter14/1
  Demux3/3 -> Saturation21/1
  Saturation22/1 -> Simulink-PS Converter15/1
  Demux3/4 -> Saturation22/1
  Demux3/5 -> Saturation23/1
  Saturation23/1 -> Simulink-PS Converter16/1
  Saturation25/1 -> Simulink-PS Converter12/1
  Demux3/7 -> Saturation25/1
  Demux3/6 -> Saturation24/1
  Saturation24/1 -> Simulink-PS Converter17/1
  Demux4/2 -> Saturation26/1
  Demux4/3 -> Saturation27/1
  Demux4/4 -> Saturation28/1
  Demux4/5 -> Saturation16/1
  Demux4/7 -> Saturation18/1
  Demux4/6 -> Saturation17/1
  Saturation19/1 -> Mux5/1
  Demux4/1 -> Saturation19/1
  Demux3/1 -> Saturation15/1
  Saturation15/1 -> Simulink-PS Converter19/1
  Saturation26/1 -> Mux5/2
  Saturation27/1 -> Mux5/3
  Saturation28/1 -> Mux5/4
  Saturation16/1 -> Mux5/5
  Saturation17/1 -> Mux5/6
  Saturation18/1 -> Mux5/7
  Mux5/1 -> Discrete-Time Integrator3/1
  Right Arm/1 -> Demux4/1
  PS-Simulink Converter23/1 -> Mux4/7
  Demux/3 -> Simulink-PS Converter2/1
  Selector/1 -> Discrete-Time Integrator/1
  Demux5/2 -> Simulink-PS Converter13/1
  Demux5/1 -> Simulink-PS Converter11/1
  dbase/1 -> Selector/1, Selector2/1, Selector1/1
  Selector2/1 -> Demux2/1
  Mux6/1 -> q_torso/1
  PS-Simulink Converter15/1 -> Mux6/3
  PS-Simulink Converter10/1 -> Mux6/2
  Selector1/1 -> Scope/1, Demux5/1
  connections:
  Solver Configuration/RConn1 -- Base Motion/LConn1 -- World Frame/RConn1 -- Mechanism Configuration/RConn1 -- Transform Sensor/LConn1
  PS-Simulink Converter5/LConn1 -- PowerBall2_1/RConn2
  PS-Simulink Converter7/LConn1 -- PowerBall3/RConn2
  Simulink-PS Converter3/RConn1 -- PowerBall1_2/LConn2
  Simulink-PS Converter9/RConn1 -- DL100/LConn2
  Simulink-PS Converter4/RConn1 -- PowerBall2/LConn2
  Simulink-PS Converter5/RConn1 -- PowerBall2_1/LConn2
  PS-Simulink Converter/LConn1 -- PowerBall1/RConn2
  PS-Simulink Converter3/LConn1 -- PowerBall1_2/RConn2
  PS-Simulink Converter4/LConn1 -- PowerBall2/RConn2
  Simulink-PS Converter8/RConn1 -- PowerBall1/LConn2
  Simulink-PS Converter6/RConn1 -- PowerBall3/LConn2
  DL100/RConn1 -- base_1_RIGID/LConn1
  DL100/RConn2 -- PS-Simulink Converter8/LConn1
  PS-Simulink Converter9/LConn1 -- PowerBall3_1/RConn2
  PowerBall1/RConn1 -- upperarm_1_RIGID/LConn1
  Simulink-PS Converter10/RConn1 -- PowerBall3_1/LConn2
  PowerBall1/LConn1 -- base_1_RIGID/RConn1
  Base1/RConn1 -- Base Motion/RConn1 -- Rigid Transform2/LConn1
  PowerBall1_2/LConn1 -- upperarm_1_RIGID/RConn1
  PowerBall1_2/RConn1 -- upperarm_1_RIGID1/LConn1
  PowerBall2/LConn1 -- upperarm_1_RIGID1/RConn1
  PowerBall2/RConn1 -- upperarm_1_RIGID2/LConn1
  PowerBall2_1/LConn1 -- upperarm_1_RIGID2/RConn1
  upperarm_1_RIGID3/LConn1 -- PowerBall2_1/RConn1
  PowerBall3/LConn1 -- upperarm_1_RIGID3/RConn1
  PowerBall3/RConn1 -- upperarm_1_RIGID4/LConn1
  PowerBall3_1/LConn1 -- upperarm_1_RIGID4/RConn1
  PowerBall3_1/RConn1 -- upperarm_1_RIGID5/LConn1
  upperarm_1_RIGID5/RConn1 -- Transform Sensor/RConn1 -- upperarm_1_RIGID6/LConn1
  PS-Simulink Converter11/LConn1 -- Transform Sensor/RConn2
  Transform Sensor/RConn3 -- PS-Simulink Converter12/LConn1
  Transform Sensor/RConn4 -- PS-Simulink Converter13/LConn1
  Base Motion/LConn2 -- Simulink-PS Converter7/RConn1
  Base Motion/LConn3 -- Simulink-PS Converter1/RConn1
  Simulink-PS Converter2/RConn1 -- Base Motion/LConn4
  Base Motion/RConn2 -- PS-Simulink Converter6/LConn1
  Base Motion/RConn3 -- PS-Simulink Converter1/LConn1
  PS-Simulink Converter2/LConn1 -- Base Motion/RConn4
  upperarm_1_RIGID12/RConn1 -- upperarm_1_RIGID13/LConn1
  Simulink-PS Converter18/RConn1 -- PowerBall4/LConn2
  PowerBall6/RConn1 -- upperarm_1_RIGID11/LConn1
  PowerBall4/LConn1 -- base_1_RIGID1/RConn1
  PS-Simulink Converter14/LConn1 -- PowerBall4/RConn2
  PowerBall1_1/LConn1 -- upperarm_1_RIGID7/RConn1
  Simulink-PS Converter14/RConn1 -- PowerBall1_1/LConn2
  PS-Simulink Converter21/LConn1 -- PowerBall6/RConn2
  PowerBall6/LConn1 -- upperarm_1_RIGID10/RConn1
  Simulink-PS Converter19/RConn1 -- DL1/LConn2
  PowerBall1_1/RConn1 -- upperarm_1_RIGID8/LConn1
  Simulink-PS Converter15/RConn1 -- PowerBall5/LConn2
  PowerBall3_2/LConn1 -- upperarm_1_RIGID11/RConn1
  PS-Simulink Converter19/LConn1 -- PowerBall5/RConn2
  PS-Simulink Converter20/LConn1 -- PowerBall2_2/RConn2
  PS-Simulink Converter18/LConn1 -- PowerBall1_1/RConn2
  upperarm_1_RIGID10/LConn1 -- PowerBall2_2/RConn1
  DL1/RConn2 -- PS-Simulink Converter22/LConn1
  PowerBall3_2/RConn1 -- upperarm_1_RIGID12/LConn1
  Simulink-PS Converter16/RConn1 -- PowerBall2_2/LConn2
  PS-Simulink Converter23/LConn1 -- PowerBall3_2/RConn2
  DL1/RConn1 -- base_1_RIGID1/LConn1
  PowerBall5/LConn1 -- upperarm_1_RIGID8/RConn1
  Simulink-PS Converter12/RConn1 -- PowerBall3_2/LConn2
  PowerBall5/RConn1 -- upperarm_1_RIGID9/LConn1
  PowerBall4/RConn1 -- upperarm_1_RIGID7/LConn1
  PowerBall2_2/LConn1 -- upperarm_1_RIGID9/RConn1
  Simulink-PS Converter17/RConn1 -- PowerBall6/LConn2
  Rigid Transform1/RConn1 -- DL1/LConn1
  Rigid Transform2/RConn1 -- Torso_Joint2/LConn1
  Rigid Transform3/LConn1 -- Torso_Joint2/RConn1
  Rigid Transform4/LConn1 -- Rigid Transform5/LConn1 -- Rigid Transform1/LConn1 -- Torso_Joint3/RConn1
  Torso_Joint3/LConn1 -- Rigid Transform3/RConn1
  Rigid Transform4/RConn1 -- DL100/LConn1
  Torso/RConn1 -- Rigid Transform5/RConn1
  Simulink-PS Converter11/RConn1 -- Torso_Joint2/LConn2
  Simulink-PS Converter13/RConn1 -- Torso_Joint3/LConn2
  PS-Simulink Converter15/LConn1 -- Torso_Joint3/RConn2
  PS-Simulink Converter10/LConn1 -- Torso_Joint2/RConn2

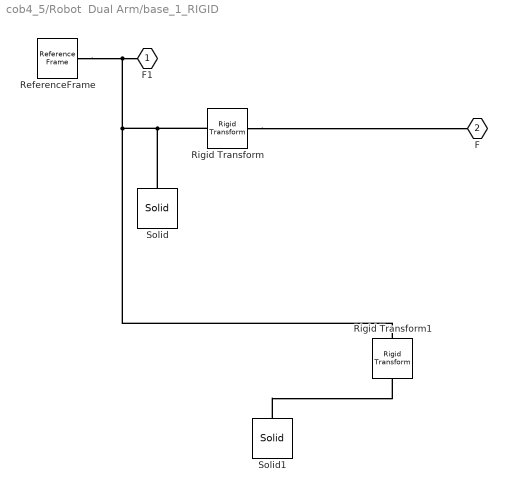
== system cob4_5/Robot  Dual Arm/base_1_RIGID ==
  ReferenceFrame : sm_lib/Frames and Transforms/Reference Frame
  Rigid Transform : sm_lib/Frames and Transforms/Rigid Transform  TranslationMethod=Cartesian  TranslationLengthUnit=m  TranslationStandardAxis=+Z  TranslationStandardOffset=max(a(1:3,4,1))  TranslationCartesianOffset=a(1:3,4,5+j)  TranslationROffset=0  TranslationROffsetUnits=m  TranslationZOffset=0  TranslationZOffsetUnits=m  TranslationThetaOffset=0  TranslationThetaOffsetUnits=deg  RotationMethod=RotationMatrix  RotationAngleUnits=deg  RotationStandardAxis=+Z  RotationAngle=0.0  RotationArbitraryAxis=[0 0 1]  FollAlignAxisA=+X  BaseAlignAxisA=+Y  FollAlignAxisB=+Y  BaseAlignAxisB=+Z  RotationSequenceAxes=FollowerAxes  RotationSequence=XYX  RotationSequenceAngles=[0 0 0]  RotationSequenceAnglesUnits=deg  RotationMatrix=a(1:3,1:3,5+j)
  Rigid Transform1 : sm_lib/Frames and Transforms/Rigid Transform  TranslationMethod=Cartesian  TranslationLengthUnit=m  TranslationStandardAxis=+Z  TranslationStandardOffset=max(a(1:3,4,3))  TranslationCartesianOffset=shoulder1_link(1:3,4,1)  TranslationROffset=0  TranslationROffsetUnits=m  TranslationZOffset=0  TranslationZOffsetUnits=m  TranslationThetaOffset=0  TranslationThetaOffsetUnits=deg  RotationMethod=RotationMatrix  RotationAngleUnits=deg  RotationStandardAxis=+Z  RotationAngle=0.0  RotationArbitraryAxis=[0 0 1]  FollAlignAxisA=+X  BaseAlignAxisA=+Y  FollAlignAxisB=+Y  BaseAlignAxisB=+Z  RotationSequenceAxes=FollowerAxes  RotationSequence=XYX  RotationSequenceAngles=[0 0 0]  RotationSequenceAnglesUnits=deg  RotationMatrix=shoulder1_link(1:3,1:3,1)
  Solid : sm_lib/Body Elements/Solid  InertiaType=PointMass  Mass=1  MassUnits=kg  CenterOfMass=[0 0 0]  CenterOfMassUnits=m  MomentsOfInertia=[1 1 1]  MomentsOfInertiaUnits=kg*m^2  ProductsOfInertia=[0 0 0]  ProductsOfInertiaUnits=kg*m^2  DensityBased=on  Density=1000  DensityUnits=kg/(m^3)  DoExposeReferenceFrame=on  SerializedFrames=<Frames/>  GraphicType=FromGeometry  MarkerShape=Sphere  MarkerSize=10  GraphicVisPropType=SimpleVisualProperties  GraphicDiffuseColor=[0.5 0.5 0.5]  GraphicSpecularColor=[0.5 0.5 0.5 1.0]  GraphicAmbientColor=[0.15 0.15 0.15 1.0]  GraphicEmissiveColor=[0.0 0.0 0.0 1.0]  GraphicShininess=75  GraphicOpacity=1.0  GeometryShape=FromFile  RectangleSize=[1 1]  RectangleSizeUnits=m  BrickDimensions=[1 1 1]  BrickDimensionUnits=m  CylinderRadius=1  CylinderRadiusUnits=m  CylinderLength=1  CylinderLengthUnits=m  SphereRadius=1  SphereRadiusUnits=m  EllipsoidRadii=[1 1 1]  EllipsoidRadiiUnits=m  ExtrusionCrossSection=[1 1; -1 1; -1 -1; 1 -1]  ExtrusionCrossSectionUnits=m  ExtrusionLength=1  ExtrusionLengthUnits=m  PolygonNumSides=3  PolygonOuterRadius=1  PolygonOuterRadiusUnits=m  ExtGeomFileType=STL  ExtGeomFileName=/home/bbrito/catkin_ws/src/schunk_modular_robotics/schunk_description/meshes/lwa4p_extended/arm_base_link.stl  ExtGeomFileUnits=m  RevolutionCrossSection=[1 1; 1 -1; 2 -1; 2 1]  RevolutionCrossSectionUnits=m  RevolutionExtent=Full  RevolutionAngle=180  RevolutionAngleUnits=deg
  Solid1 : sm_lib/Body Elements/Solid  InertiaType=Custom  Mass=3.9  MassUnits=kg  CenterOfMass=[18 0 82]  CenterOfMassUnits=mm  MomentsOfInertia=[0.0378 0.042799 0.010997]  MomentsOfInertiaUnits=kg*m^2  ProductsOfInertia=[0.00978 0.0133 0.00978]  ProductsOfInertiaUnits=kg*m^2  DensityBased=on  Density=1000  DensityUnits=kg/(m^3)  DoExposeReferenceFrame=on  SerializedFrames=<Frames/>  GraphicType=FromGeometry  MarkerShape=Sphere  MarkerSize=10  GraphicVisPropType=SimpleVisualProperties  GraphicDiffuseColor=[0.5 0.5 0.5]  GraphicSpecularColor=[0.5 0.5 0.5 1.0]  GraphicAmbientColor=[0.15 0.15 0.15 1.0]  GraphicEmissiveColor=[0.0 0.0 0.0 1.0]  GraphicShininess=75  GraphicOpacity=1.0  GeometryShape=FromFile  RectangleSize=[1 1]  RectangleSizeUnits=m  BrickDimensions=[1 1 1]  BrickDimensionUnits=m  CylinderRadius=1  CylinderRadiusUnits=m  CylinderLength=1  CylinderLengthUnits=m  SphereRadius=1  SphereRadiusUnits=m  EllipsoidRadii=[1 1 1]  EllipsoidRadiiUnits=m  ExtrusionCrossSection=[1 1; -1 1; -1 -1; 1 -1]  ExtrusionCrossSectionUnits=m  ExtrusionLength=1  ExtrusionLengthUnits=m  PolygonNumSides=3  PolygonOuterRadius=1  PolygonOuterRadiusUnits=m  ExtGeomFileType=STL  ExtGeomFileName=/home/bbrito/schunk_sim/lwa4p/arm_11_link.stl  ExtGeomFileUnits=m  RevolutionCrossSection=[1 1; 1 -1; 2 -1; 2 1]  RevolutionCrossSectionUnits=m  RevolutionExtent=Full  RevolutionAngle=180  RevolutionAngleUnits=deg
  F1 : PMIOPort  Port=1  Side=Left
  F : PMIOPort  Port=2  Side=Right
  connections:
  F1/RConn1 -- Rigid Transform1/LConn1 -- Rigid Transform/LConn1 -- Solid/RConn1 -- ReferenceFrame/RConn1
  Rigid Transform/RConn1 -- F/RConn1
  Solid1/RConn1 -- Rigid Transform1/RConn1

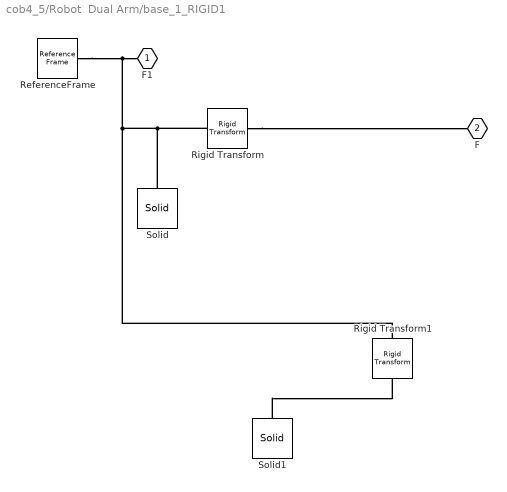
== system cob4_5/Robot  Dual Arm/base_1_RIGID1 ==
  ReferenceFrame : sm_lib/Frames and Transforms/Reference Frame
  Rigid Transform : sm_lib/Frames and Transforms/Rigid Transform  TranslationMethod=Cartesian  TranslationLengthUnit=m  TranslationStandardAxis=+Z  TranslationStandardOffset=max(a(1:3,4,1))  TranslationCartesianOffset=a2(1:3,4,2)  TranslationROffset=0  TranslationROffsetUnits=m  TranslationZOffset=0  TranslationZOffsetUnits=m  TranslationThetaOffset=0  TranslationThetaOffsetUnits=deg  RotationMethod=RotationMatrix  RotationAngleUnits=deg  RotationStandardAxis=+Z  RotationAngle=0.0  RotationArbitraryAxis=[0 0 1]  FollAlignAxisA=+X  BaseAlignAxisA=+Y  FollAlignAxisB=+Y  BaseAlignAxisB=+Z  RotationSequenceAxes=FollowerAxes  RotationSequence=XYX  RotationSequenceAngles=[0 0 0]  RotationSequenceAnglesUnits=deg  RotationMatrix=a2(1:3,1:3,2)
  Rigid Transform1 : sm_lib/Frames and Transforms/Rigid Transform  TranslationMethod=Cartesian  TranslationLengthUnit=m  TranslationStandardAxis=+Z  TranslationStandardOffset=max(a(1:3,4,3))  TranslationCartesianOffset=shoulder2_link(1:3,4,1)  TranslationROffset=0  TranslationROffsetUnits=m  TranslationZOffset=0  TranslationZOffsetUnits=m  TranslationThetaOffset=0  TranslationThetaOffsetUnits=deg  RotationMethod=RotationMatrix  RotationAngleUnits=deg  RotationStandardAxis=+Z  RotationAngle=0.0  RotationArbitraryAxis=[0 0 1]  FollAlignAxisA=+X  BaseAlignAxisA=+Y  FollAlignAxisB=+Y  BaseAlignAxisB=+Z  RotationSequenceAxes=FollowerAxes  RotationSequence=XYX  RotationSequenceAngles=[0 0 0]  RotationSequenceAnglesUnits=deg  RotationMatrix=shoulder2_link(1:3,1:3,1)
  Solid : sm_lib/Body Elements/Solid  InertiaType=PointMass  Mass=1  MassUnits=kg  CenterOfMass=[0 0 0]  CenterOfMassUnits=m  MomentsOfInertia=[1 1 1]  MomentsOfInertiaUnits=kg*m^2  ProductsOfInertia=[0 0 0]  ProductsOfInertiaUnits=kg*m^2  DensityBased=on  Density=1000  DensityUnits=kg/(m^3)  DoExposeReferenceFrame=on  SerializedFrames=<Frames/>  GraphicType=FromGeometry  MarkerShape=Sphere  MarkerSize=10  GraphicVisPropType=SimpleVisualProperties  GraphicDiffuseColor=[0.5 0.5 0.5]  GraphicSpecularColor=[0.5 0.5 0.5 1.0]  GraphicAmbientColor=[0.15 0.15 0.15 1.0]  GraphicEmissiveColor=[0.0 0.0 0.0 1.0]  GraphicShininess=75  GraphicOpacity=1.0  GeometryShape=FromFile  RectangleSize=[1 1]  RectangleSizeUnits=m  BrickDimensions=[1 1 1]  BrickDimensionUnits=m  CylinderRadius=1  CylinderRadiusUnits=m  CylinderLength=1  CylinderLengthUnits=m  SphereRadius=1  SphereRadiusUnits=m  EllipsoidRadii=[1 1 1]  EllipsoidRadiiUnits=m  ExtrusionCrossSection=[1 1; -1 1; -1 -1; 1 -1]  ExtrusionCrossSectionUnits=m  ExtrusionLength=1  ExtrusionLengthUnits=m  PolygonNumSides=3  PolygonOuterRadius=1  PolygonOuterRadiusUnits=m  ExtGeomFileType=STL  ExtGeomFileName=/home/bbrito/catkin_ws/src/schunk_modular_robotics/schunk_description/meshes/lwa4p_extended/arm_base_link.stl  ExtGeomFileUnits=m  RevolutionCrossSection=[1 1; 1 -1; 2 -1; 2 1]  RevolutionCrossSectionUnits=m  RevolutionExtent=Full  RevolutionAngle=180  RevolutionAngleUnits=deg
  Solid1 : sm_lib/Body Elements/Solid  InertiaType=Custom  Mass=3.9  MassUnits=kg  CenterOfMass=[18 0 82]  CenterOfMassUnits=mm  MomentsOfInertia=[0.0378 0.042799 0.010997]  MomentsOfInertiaUnits=kg*m^2  ProductsOfInertia=[0.00978 0.0133 0.00978]  ProductsOfInertiaUnits=kg*m^2  DensityBased=on  Density=1000  DensityUnits=kg/(m^3)  DoExposeReferenceFrame=on  SerializedFrames=<Frames/>  GraphicType=FromGeometry  MarkerShape=Sphere  MarkerSize=10  GraphicVisPropType=SimpleVisualProperties  GraphicDiffuseColor=[0.5 0.5 0.5]  GraphicSpecularColor=[0.5 0.5 0.5 1.0]  GraphicAmbientColor=[0.15 0.15 0.15 1.0]  GraphicEmissiveColor=[0.0 0.0 0.0 1.0]  GraphicShininess=75  GraphicOpacity=1.0  GeometryShape=FromFile  RectangleSize=[1 1]  RectangleSizeUnits=m  BrickDimensions=[1 1 1]  BrickDimensionUnits=m  CylinderRadius=1  CylinderRadiusUnits=m  CylinderLength=1  CylinderLengthUnits=m  SphereRadius=1  SphereRadiusUnits=m  EllipsoidRadii=[1 1 1]  EllipsoidRadiiUnits=m  ExtrusionCrossSection=[1 1; -1 1; -1 -1; 1 -1]  ExtrusionCrossSectionUnits=m  ExtrusionLength=1  ExtrusionLengthUnits=m  PolygonNumSides=3  PolygonOuterRadius=1  PolygonOuterRadiusUnits=m  ExtGeomFileType=STL  ExtGeomFileName=/home/bbrito/schunk_sim/lwa4p/arm_11_link.stl  ExtGeomFileUnits=m  RevolutionCrossSection=[1 1; 1 -1; 2 -1; 2 1]  RevolutionCrossSectionUnits=m  RevolutionExtent=Full  RevolutionAngle=180  RevolutionAngleUnits=deg
  F1 : PMIOPort  Port=1  Side=Left
  F : PMIOPort  Port=2  Side=Right
  connections:
  F1/RConn1 -- Rigid Transform1/LConn1 -- Rigid Transform/LConn1 -- Solid/RConn1 -- ReferenceFrame/RConn1
  Rigid Transform/RConn1 -- F/RConn1
  Solid1/RConn1 -- Rigid Transform1/RConn1
